simulink model "TestStructure"  (R2022b)
settings: Solver=FixedStepDiscrete  StartTime=0.0  StopTime=300  FixedStep=SampleTime  RelTol=1e-3
InitFcn:
  | SampleTime = 0.001;
  | ButtonValue=0;
  | load("BusConfig.mat");
model workspace (MAT data in the model file):
  Manual_Auto = 1
  Pattern = 1
  Pause_Start = 1
  Stop = 1
  Unlock_Lock = 1
undefined symbols (not defined in the file or in its folder): DiscIntNeverNeededParam
libraries: dspfdesign x4, dspstat3 x4
(part 3 of 3)

== system TestStructure/Control/Tasks/LLBManualTask/Subsystem1/If Action Subsystem2 ==
  Motor1Pos : Inport
  Action Port : ActionPort  ActionPortLabel=if((u1 >= u2))
  Out1 : Outport
  wires:
  Motor1Pos/1 -> Out1/1

== system TestStructure/Control/Tasks/LLBManualTask/Subsystem2/If Action Subsystem4 ==
  In1 : Inport
  Action Port : ActionPort  ActionPortLabel=else
  Out1 : Outport
  wires:
  In1/1 -> Out1/1

== system TestStructure/Control/Tasks/LLBManualTask/Subsystem2/If Action Subsystem5 ==
  In1 : Inport
  Action Port : ActionPort  ActionPortLabel=if((u1 <= u2))
  Out1 : Outport
  wires:
  In1/1 -> Out1/1

== system TestStructure/Control/Tasks/LLBManualTask/Subsystem3/If Action Subsystem1 ==
  In1 : Inport
  Action Port : ActionPort  ActionPortLabel=else
  Out1 : Outport
  wires:
  In1/1 -> Out1/1

== system TestStructure/Control/Tasks/LLBManualTask/Subsystem3/If Action Subsystem2 ==
  Motor1Pos : Inport
  Action Port : ActionPort  ActionPortLabel=if((u1 >= u2))
  Out1 : Outport
  wires:
  Motor1Pos/1 -> Out1/1

== system TestStructure/Control/Tasks/LLWManualTask/Subsystem/If Action Subsystem4 ==
  In1 : Inport
  Action Port : ActionPort  ActionPortLabel=else
  Out1 : Outport
  wires:
  In1/1 -> Out1/1

== system TestStructure/Control/Tasks/LLWManualTask/Subsystem/If Action Subsystem5 ==
  In1 : Inport
  Action Port : ActionPort  ActionPortLabel=if((u1 <= u2))
  Out1 : Outport
  wires:
  In1/1 -> Out1/1

== system TestStructure/Control/Tasks/LLWManualTask/Subsystem1/If Action Subsystem1 ==
  In1 : Inport
  Action Port : ActionPort  ActionPortLabel=else
  Out1 : Outport
  wires:
  In1/1 -> Out1/1

== system TestStructure/Control/Tasks/LLWManualTask/Subsystem1/If Action Subsystem2 ==
  Motor1Pos : Inport
  Action Port : ActionPort  ActionPortLabel=if((u1 >= u2))
  Out1 : Outport
  wires:
  Motor1Pos/1 -> Out1/1

== system TestStructure/Control/Tasks/LLWManualTask/Subsystem2/If Action Subsystem4 ==
  In1 : Inport
  Action Port : ActionPort  ActionPortLabel=else
  Out1 : Outport
  wires:
  In1/1 -> Out1/1

== system TestStructure/Control/Tasks/LLWManualTask/Subsystem2/If Action Subsystem5 ==
  In1 : Inport
  Action Port : ActionPort  ActionPortLabel=if((u1 <= u2))
  Out1 : Outport
  wires:
  In1/1 -> Out1/1

== system TestStructure/Control/Tasks/LLWManualTask/Subsystem3/If Action Subsystem1 ==
  In1 : Inport
  Action Port : ActionPort  ActionPortLabel=else
  Out1 : Outport
  wires:
  In1/1 -> Out1/1

== system TestStructure/Control/Tasks/LLWManualTask/Subsystem3/If Action Subsystem2 ==
  Motor1Pos : Inport
  Action Port : ActionPort  ActionPortLabel=if((u1 >= u2))
  Out1 : Outport
  wires:
  Motor1Pos/1 -> Out1/1

== stateflow chart TestStructure/Control/Tasks/LLBManualTask/RythmModel/Chart ==
  state IntStateOperation
    Count =1/(Period*SampleTime);
    Input=1/Period;
    Reset = 0;
  state ResetOperation
    Reset = 1;
  (default) -> IntStateOperation
  ResetOperation -> IntStateOperation : [IntVal<(Count)*(Period*SampleTime)]
  IntStateOperation -> ResetOperation : [IntVal>=(Count)*(Period*SampleTime)||(ResetState==1)]
  data: ResetState input; Period input; SampleTime input; Input output; Reset output; IntVal input; Count local

== stateflow chart TestStructure/Control/Tasks/LLWManualTask/RythmModel/Chart ==
  state IntStateOperation
    Count =1/(Period*SampleTime);
    Input=1/Period;
    Reset = 0;
  state ResetOperation
    Reset = 1;
  (default) -> IntStateOperation
  ResetOperation -> IntStateOperation : [IntVal<(Count)*(Period*SampleTime)]
  IntStateOperation -> ResetOperation : [IntVal>=(Count)*(Period*SampleTime)||(ResetState==1)]
  data: ResetState input; Period input; SampleTime input; Input output; Reset output; IntVal input; Count local

== stateflow chart TestStructure/Control/PanelController/ControlPannelStateMachine ==
  state Pause
    State = "Pause";
    if(Pause_StartButtonPressed==0)
    Pause_StartButtonPressed_temp = 0;
    end
  state Stop
    (history)
    state Stop
      State = "Stop";
    state LowerLimb_Follow
      state LowerLimb_Follow
        if(PatternButtonPressed==0)
        PatternButtonPressed_temp = 0;
        end
        State = "Stop";
        Mode = "Lower_Limb_Follow";
        ManualAuto = "";
      (default) -> Stop.LowerLimb_Follow.LowerLimb_Follow
    state LowerLimb_FlutterKick
      (history)
      state LowerLimb_FlutterKick
        if(PatternButtonPressed==0)
        PatternButtonPressed_temp = 0;
        end
        State = "Stop";
        Mode = "Lower_Limb_FlutterKick";
      state LLFK_Manual_Torque
        if(PatternButtonPressed==0)
        PatternButtonPressed_temp = 0;
        end
        if(Manual_AutoButtonPressed==0)
        Manual_AutoButtonPressed_temp = 0;
        end
        State = "Stop";
        Mode = "Lower_Limb_FlutterKick";
        ManualAuto = "LLFK_Manual_Torque";
      state LLFK_Manual_Freq
        if(PatternButtonPressed==0)
        PatternButtonPressed_temp = 0;
        end
        if(Manual_AutoButtonPressed==0)
        Manual_AutoButtonPressed_temp = 0;
        end
        State = "Stop";
        Mode = "Lower_Limb_FlutterKick";
        ManualAuto = "LLFK_Manual_Freq";
      state LLFK_Manual_Pos
        if(PatternButtonPressed==0)
        PatternButtonPressed_temp = 0;
        end
        if(Manual_AutoButtonPressed==0)
        Manual_AutoButtonPressed_temp = 0;
        end
        State = "Stop";
        Mode = "Lower_Limb_FlutterKick";
        ManualAuto = "LLFK_Manual_Pos";
      state LLFK_Auto
        if(PatternButtonPressed==0)
        PatternButtonPressed_temp = 0;
        end
        if(Manual_AutoButtonPressed==0)
        Manual_AutoButtonPressed_temp = 0;
        end
        State = "Stop";
        Mode = "Lower_Limb_FlutterKick";
        ManualAuto = "LLFK_Auto";
      (default) -> Stop.LowerLimb_FlutterKick.LowerLimb_FlutterKick
      Stop.LowerLimb_FlutterKick.LowerLimb_FlutterKick -> LLFK_Manual_Freq
      LLFK_Manual_Freq -> LLFK_Manual_Torque : [(Manual_AutoButtonPressed_temp==0)&&(Manual_AutoButtonPressed>0)]{Manual_AutoButtonPressed_temp=1;}
      LLFK_Manual_Torque -> LLFK_Manual_Pos : [(Manual_AutoButtonPressed_temp==0)&&(Manual_AutoButtonPressed>0)]{Manual_AutoButtonPressed_temp=1;}
      LLFK_Auto -> LLFK_Manual_Freq : [(Manual_AutoButtonPressed_temp==0)&&(Manual_AutoButtonPressed>0)]{Manual_AutoButtonPressed_temp=1;}
      LLFK_Manual_Pos -> LLFK_Auto : [(Manual_AutoButtonPressed_temp==0)&&(Manual_AutoButtonPressed>0)]{Manual_AutoButtonPressed_temp=1;}
    state LowerLimb_Breaststroke
      (history)
      state Lower_Limb_Breaststroke
        if(PatternButtonPressed==0)
        PatternButtonPressed_temp = 0;
        end
        State = "Stop";
        Mode = "Lower_Limb_Breaststroke";
      state LLB_Manual_Torque
        if(PatternButtonPressed==0)
        PatternButtonPressed_temp = 0;
        end
        if(Manual_AutoButtonPressed==0)
        Manual_AutoButtonPressed_temp = 0;
        end
        State = "Stop";
        Mode = "Lower_Limb_Breaststroke";
        ManualAuto = "LLB_Manual_Torque";
      state LLB_Manual_Freq
        if(PatternButtonPressed==0)
        PatternButtonPressed_temp = 0;
        end
        if(Manual_AutoButtonPressed==0)
        Manual_AutoButtonPressed_temp = 0;
        end
        State = "Stop";
        Mode = "Lower_Limb_Breaststroke";
        ManualAuto = "LLB_Manual_Freq";
      state LLB_Manual_Pos
        if(PatternButtonPressed==0)
        PatternButtonPressed_temp = 0;
        end
        if(Manual_AutoButtonPressed==0)
        Manual_AutoButtonPressed_temp = 0;
        end
        State = "Stop";
        Mode = "Lower_Limb_Breaststroke";
        ManualAuto = "LLB_Manual_Pos";
      state LLB_Auto
        if(PatternButtonPressed==0)
        PatternButtonPressed_temp = 0;
        end
        if(Manual_AutoButtonPressed==0)
        Manual_AutoButtonPressed_temp = 0;
        end
        State = "Stop";
        Mode = "Lower_Limb_Breaststroke";
        ManualAuto = "LLB_Auto";
      (default) -> Lower_Limb_Breaststroke
      Lower_Limb_Breaststroke -> LLB_Manual_Freq
      LLB_Manual_Freq -> LLB_Manual_Torque : [(Manual_AutoButtonPressed_temp==0)&&(Manual_AutoButtonPressed>0)]{Manual_AutoButtonPressed_temp=1;}
      LLB_Manual_Torque -> LLB_Manual_Pos : [(Manual_AutoButtonPressed_temp==0)&&(Manual_AutoButtonPressed>0)]{Manual_AutoButtonPressed_temp=1;}
      LLB_Auto -> LLB_Manual_Freq : [(Manual_AutoButtonPressed_temp==0)&&(Manual_AutoButtonPressed>0)]{Manual_AutoButtonPressed_temp=1;}
      LLB_Manual_Pos -> LLB_Auto : [(Manual_AutoButtonPressed_temp==0)&&(Manual_AutoButtonPressed>0)]{Manual_AutoButtonPressed_temp=1;}
    state LowerLimb_Walk
      (history)
      state LowerLimb_Walk
        if(PatternButtonPressed==0)
        PatternButtonPressed_temp = 0;
        end
        State = "Stop";
        Mode = "Lower_Limb_Walk";
      state LLW_Manual_Torque
        if(PatternButtonPressed==0)
        PatternButtonPressed_temp = 0;
        end
        if(Manual_AutoButtonPressed==0)
        Manual_AutoButtonPressed_temp = 0;
        end
        State = "Stop";
        Mode = "Lower_Limb_Walk";
        ManualAuto = "LLW_Manual_Torque";
      state LLW_Manual_Freq
        if(PatternButtonPressed==0)
        PatternButtonPressed_temp = 0;
        end
        if(Manual_AutoButtonPressed==0)
        Manual_AutoButtonPressed_temp = 0;
        end
        State = "Stop";
        Mode = "Lower_Limb_Walk";
        ManualAuto = "LLW_Manual_Freq";
      state LLW_Manual_Pos
        if(PatternButtonPressed==0)
        PatternButtonPressed_temp = 0;
        end
        if(Manual_AutoButtonPressed==0)
        Manual_AutoButtonPressed_temp = 0;
        end
        State = "Stop";
        Mode = "Lower_Limb_Walk";
        ManualAuto = "LLW_Manual_Pos";
      state LLW_Auto
        if(PatternButtonPressed==0)
        PatternButtonPressed_temp = 0;
        end
        if(Manual_AutoButtonPressed==0)
        Manual_AutoButtonPressed_temp = 0;
        end
        State = "Stop";
        Mode = "Lower_Limb_Walk";
        ManualAuto = "LLW_Auto";
      (default) -> Stop.LowerLimb_Walk.LowerLimb_Walk
      Stop.LowerLimb_Walk.LowerLimb_Walk -> LLW_Manual_Freq
      LLW_Manual_Freq -> LLW_Manual_Torque : [(Manual_AutoButtonPressed_temp==0)&&(Manual_AutoButtonPressed>0)]{Manual_AutoButtonPressed_temp=1;}
      LLW_Manual_Torque -> LLW_Manual_Pos : [(Manual_AutoButtonPressed_temp==0)&&(Manual_AutoButtonPressed>0)]{Manual_AutoButtonPressed_temp=1;}
      LLW_Auto -> LLW_Manual_Freq : [(Manual_AutoButtonPressed_temp==0)&&(Manual_AutoButtonPressed>0)]{Manual_AutoButtonPressed_temp=1;}
      LLW_Manual_Pos -> LLW_Auto : [(Manual_AutoButtonPressed_temp==0)&&(Manual_AutoButtonPressed>0)]{Manual_AutoButtonPressed_temp=1;}
    (default) -> Stop.Stop
    Stop.Stop -> Stop.LowerLimb_Follow
    Stop.LowerLimb_Follow -> Stop.LowerLimb_FlutterKick : [(PatternButtonPressed_temp==0)&&(PatternButtonPressed>0)]{PatternButtonPressed_temp=1;}
    LowerLimb_Breaststroke -> Stop.LowerLimb_Walk : [(PatternButtonPressed_temp==0)&&(PatternButtonPressed>0)]{PatternButtonPressed_temp=1;}
    Stop.LowerLimb_FlutterKick -> LowerLimb_Breaststroke : [(PatternButtonPressed_temp==0)&&(PatternButtonPressed>0)]{PatternButtonPressed_temp=1;}
    Stop.LowerLimb_Walk -> Stop.LowerLimb_Follow : [(PatternButtonPressed_temp==0)&&(PatternButtonPressed>0)]{PatternButtonPressed_temp=1;}
  state Start
    state Start
      State = "Start";
      if(Pause_StartButtonPressed==0)
      Pause_StartButtonPressed_temp = 0;
      end
    state UpperLimb_Lock
      if(Pause_StartButtonPressed==0)
      Pause_StartButtonPressed_temp = 0;
      end
      if(Unlock_LockButtonPressed==0)
      Unlock_LockButtonPressed_temp = 0;
      end
      State = "Start";
      UnlockLock = "UpperLimb_Lock";
    state UpperLimb_UnLock
      if(Pause_StartButtonPressed==0)
      Pause_StartButtonPressed_temp = 0;
      end
      if(Unlock_LockButtonPressed==0)
      Unlock_LockButtonPressed_temp = 0;
      end
      State = "Start";
      UnlockLock = "UpperLimb_Unlock";
    (default) -> Start.Start
    Start.Start -> UpperLimb_UnLock
    UpperLimb_Lock -> UpperLimb_UnLock : [(Unlock_LockButtonPressed_temp==0)&&(Unlock_LockButtonPressed>0)]{Unlock_LockButtonPressed_temp=1;}
    UpperLimb_UnLock -> UpperLimb_Lock : [(Unlock_LockButtonPressed_temp==0)&&(Unlock_LockButtonPressed>0)]{Unlock_LockButtonPressed_temp=1;}
  Start -> Pause : [(Pause_StartButtonPressed_temp==0)&&(Pause_StartButtonPressed>0)]{Pause_StartButtonPressed_temp=1;UnlockLock = "UpperLimb_Unlock";}
  Pause -> Stop [order 2] : [StopButtonPressed>0]
  Pause -> Start [order 1] : [(Pause_StartButtonPressed_temp==0)&&(Pause_StartButtonPressed>0)&&(TaskFinished==9)]{Pause_StartButtonPressed_temp=1;}
  (default) -> Stop
  Stop -> Start : [(Pause_StartButtonPressed>0)&&(TaskFinished==1)]{Pause_StartButtonPressed_temp=1;}
  data: TaskFinished input; StopButtonPressed input; State output; Pause_StartButtonPressed input; Pause_StartButtonPressed_temp local; PatternButtonPressed input; Manual_AutoButtonPressed input; Manual_AutoButtonPressed_temp local; PatternButtonPressed_temp local; Mode output string; ManualAuto output string; UnlockLock output string; Unlock_LockButtonPressed input; Unlock_LockButtonPressed_temp local

== stateflow chart TestStructure/Control/PanelController/KnobStateMachine ==
  state Start
    kState = "Start";
  state Adjust
    state LLF_Adjust
    state Adjust
      kState = "Adjust";
    state LLFK_Adjust
      state LLFK_Auto
      state LLFK_Adjust
        kState = "LLFK_Adjust";
      state LLFK_Freq_Adjust
        state LLFK_Freq_Adjust
          kState = "LLFK_Freq";
          LLFK_Freq = 0;
          LLFK_Torque_Up = 0;
          LLFK_Torque_Down = 0;
          LLFK_Pos_Up = 0;
          LLFK_Pos_Down = 0;
          LLB_Freq = 0;
          LLB_Torque_Up = 0;
          LLB_Torque_Down = 0;
          LLB_Pos_Up = 0;
          LLB_Pos_Down = 0;
          LLW_Freq = 0;
          LLW_Torque_Up = 0;
          LLW_Torque_Down = 0;
          LLW_Pos_Up = 0;
          LLW_Pos_Down = 0;
          Freq_Up_temp = 0;
          Freq_Down_temp = 0;
        state Freq_Up
          if(Freq_Up==0)
          Freq_Up_temp = 0;
          LLFK_Freq = 1;
          end
        state Freq_Down
          if(Freq_Down==0)
          Freq_Down_temp = 0;
          LLFK_Freq = -1;
          end
        (default) -> Adjust.LLFK_Adjust.LLFK_Freq_Adjust.LLFK_Freq_Adjust
        Adjust.LLFK_Adjust.LLFK_Freq_Adjust.LLFK_Freq_Adjust -> Adjust.LLFK_Adjust.LLFK_Freq_Adjust.Freq_Down [order 2] : [(Freq_Down_temp==0)&&(Freq_Down>0)]{Freq_Down_temp=1;}
        Adjust.LLFK_Adjust.LLFK_Freq_Adjust.LLFK_Freq_Adjust -> Adjust.LLFK_Adjust.LLFK_Freq_Adjust.Freq_Up [order 1] : [(Freq_Up_temp==0)&&(Freq_Up>0)]{Freq_Up_temp=1;}
        Adjust.LLFK_Adjust.LLFK_Freq_Adjust.Freq_Up -> Adjust.LLFK_Adjust.LLFK_Freq_Adjust.LLFK_Freq_Adjust : [Freq_Up_temp == 0]
        Adjust.LLFK_Adjust.LLFK_Freq_Adjust.Freq_Down -> Adjust.LLFK_Adjust.LLFK_Freq_Adjust.LLFK_Freq_Adjust : [Freq_Down_temp == 0]
      state LLFK_Torque_Adjust
        state Negtive_Up
          if(Negtive_Up==0)
          Negtive_Up_temp = 0;
          LLFK_Torque_Down = 1;
          end
        state LLFK_Torque_Adjust
          kState = "LLFK_Torq";
          LLFK_Freq = 0;
          LLFK_Torque_Up = 0;
          LLFK_Torque_Down = 0;
          LLFK_Pos_Up = 0;
          LLFK_Pos_Down = 0;
          LLB_Freq = 0;
          LLB_Torque_Up = 0;
          LLB_Torque_Down = 0;
          LLB_Pos_Up = 0;
          LLB_Pos_Down = 0;
          LLW_Freq = 0;
          LLW_Torque_Up = 0;
          LLW_Torque_Down = 0;
          LLW_Pos_Up = 0;
          LLW_Pos_Down = 0;
          Negtive_Up_temp = 0;
          Negtive_Down_temp = 0;
          Positive_Up_temp = 0;
          Positive_Down_temp = 0;
        state Negtive_Down
          if(Negtive_Down==0)
          Negtive_Down_temp = 0;
          LLFK_Torque_Down = -1;
          end
        state Positive_Up
          if(Positive_Up==0)
          Positive_Up_temp = 0;
          LLFK_Torque_Up = 1;
          end
        state Positive_Down
          if(Positive_Down==0)
          Positive_Down_temp = 0;
          LLFK_Torque_Up = -1;
          end
        (default) -> Adjust.LLFK_Adjust.LLFK_Torque_Adjust.LLFK_Torque_Adjust
        Adjust.LLFK_Adjust.LLFK_Torque_Adjust.LLFK_Torque_Adjust -> Adjust.LLFK_Adjust.LLFK_Torque_Adjust.Negtive_Up [order 4] : [(Negtive_Up_temp==0)&&(Negtive_Up>0)]{Negtive_Up_temp=1;}
        Adjust.LLFK_Adjust.LLFK_Torque_Adjust.LLFK_Torque_Adjust -> Adjust.LLFK_Adjust.LLFK_Torque_Adjust.Negtive_Down [order 2] : [(Negtive_Down_temp==0)&&(Negtive_Down>0)]{Negtive_Down_temp=1;}
        Adjust.LLFK_Adjust.LLFK_Torque_Adjust.Negtive_Down -> Adjust.LLFK_Adjust.LLFK_Torque_Adjust.LLFK_Torque_Adjust : [Negtive_Down_temp == 0]
        Adjust.LLFK_Adjust.LLFK_Torque_Adjust.Negtive_Up -> Adjust.LLFK_Adjust.LLFK_Torque_Adjust.LLFK_Torque_Adjust : [Negtive_Up_temp == 0]
        Adjust.LLFK_Adjust.LLFK_Torque_Adjust.LLFK_Torque_Adjust -> Adjust.LLFK_Adjust.LLFK_Torque_Adjust.Positive_Up [order 3] : [(Positive_Up_temp==0)&&(Positive_Up>0)]{Positive_Up_temp=1;}
        Adjust.LLFK_Adjust.LLFK_Torque_Adjust.LLFK_Torque_Adjust -> Adjust.LLFK_Adjust.LLFK_Torque_Adjust.Positive_Down [order 1] : [(Positive_Down_temp==0)&&(Positive_Down>0)]{Positive_Down_temp=1;}
        Adjust.LLFK_Adjust.LLFK_Torque_Adjust.Positive_Up -> Adjust.LLFK_Adjust.LLFK_Torque_Adjust.LLFK_Torque_Adjust : [Positive_Up_temp == 0]
        Adjust.LLFK_Adjust.LLFK_Torque_Adjust.Positive_Down -> Adjust.LLFK_Adjust.LLFK_Torque_Adjust.LLFK_Torque_Adjust : [Positive_Down_temp == 0]
      state LLFK_Pos_Adjust
        state Negtive_Up
          if(Negtive_Up==0)
          Negtive_Up_temp = 0;
          LLFK_Pos_Down = 1;
          end
        state LLFK_Pos_Adjust
          kState = "LLFK_Pos";
          LLFK_Freq = 0;
          LLFK_Torque_Up = 0;
          LLFK_Torque_Down = 0;
          LLFK_Pos_Up = 0;
          LLFK_Pos_Down = 0;
          LLB_Freq = 0;
          LLB_Torque_Up = 0;
          LLB_Torque_Down = 0;
          LLB_Pos_Up = 0;
          LLB_Pos_Down = 0;
          LLW_Freq = 0;
          LLW_Torque_Up = 0;
          LLW_Torque_Down = 0;
          LLW_Pos_Up = 0;
          LLW_Pos_Down = 0;
          Negtive_Up_temp = 0;
          Negtive_Down_temp = 0;
          Positive_Up_temp = 0;
          Positive_Down_temp = 0;
        state Negtive_Down
          if(Negtive_Down==0)
          Negtive_Down_temp = 0;
          LLFK_Pos_Down = -1;
          end
        state Positive_Up
          if(Positive_Up==0)
          Positive_Up_temp = 0;
          LLFK_Pos_Up = 1;
          end
        state Positive_Down
          if(Positive_Down==0)
          Positive_Down_temp = 0;
          LLFK_Pos_Up = -1;
          end
        (default) -> Adjust.LLFK_Adjust.LLFK_Pos_Adjust.LLFK_Pos_Adjust
        Adjust.LLFK_Adjust.LLFK_Pos_Adjust.LLFK_Pos_Adjust -> Adjust.LLFK_Adjust.LLFK_Pos_Adjust.Negtive_Up [order 4] : [(Negtive_Up_temp==0)&&(Negtive_Up>0)]{Negtive_Up_temp=1;}
        Adjust.LLFK_Adjust.LLFK_Pos_Adjust.LLFK_Pos_Adjust -> Adjust.LLFK_Adjust.LLFK_Pos_Adjust.Negtive_Down [order 2] : [(Negtive_Down_temp==0)&&(Negtive_Down>0)]{Negtive_Down_temp=1;}
        Adjust.LLFK_Adjust.LLFK_Pos_Adjust.Negtive_Down -> Adjust.LLFK_Adjust.LLFK_Pos_Adjust.LLFK_Pos_Adjust : [Negtive_Down_temp == 0]
        Adjust.LLFK_Adjust.LLFK_Pos_Adjust.Negtive_Up -> Adjust.LLFK_Adjust.LLFK_Pos_Adjust.LLFK_Pos_Adjust : [Negtive_Up_temp == 0]
        Adjust.LLFK_Adjust.LLFK_Pos_Adjust.LLFK_Pos_Adjust -> Adjust.LLFK_Adjust.LLFK_Pos_Adjust.Positive_Up [order 3] : [(Positive_Up_temp==0)&&(Positive_Up>0)]{Positive_Up_temp=1;}
        Adjust.LLFK_Adjust.LLFK_Pos_Adjust.LLFK_Pos_Adjust -> Adjust.LLFK_Adjust.LLFK_Pos_Adjust.Positive_Down [order 1] : [(Positive_Down_temp==0)&&(Positive_Down>0)]{Positive_Down_temp=1;}
        Adjust.LLFK_Adjust.LLFK_Pos_Adjust.Positive_Up -> Adjust.LLFK_Adjust.LLFK_Pos_Adjust.LLFK_Pos_Adjust : [Positive_Up_temp == 0]
        Adjust.LLFK_Adjust.LLFK_Pos_Adjust.Positive_Down -> Adjust.LLFK_Adjust.LLFK_Pos_Adjust.LLFK_Pos_Adjust : [Positive_Down_temp == 0]
      Adjust.LLFK_Adjust.LLFK_Adjust -> LLFK_Auto [order 4] : [ManualAuto=="LLFK_Auto"]{Display_State=1;}
      LLFK_Auto -> Adjust.LLFK_Adjust.LLFK_Adjust : [ManualAuto~="LLFK_Auto"]{Display_State=2;}
      (default) -> Adjust.LLFK_Adjust.LLFK_Adjust
      Adjust.LLFK_Adjust.LLFK_Pos_Adjust -> Adjust.LLFK_Adjust.LLFK_Adjust : [ManualAuto~="LLFK_Manual_Pos"]
      Adjust.LLFK_Adjust.LLFK_Adjust -> Adjust.LLFK_Adjust.LLFK_Freq_Adjust [order 3] : [ManualAuto=="LLFK_Manual_Freq"]
      Adjust.LLFK_Adjust.LLFK_Freq_Adjust -> Adjust.LLFK_Adjust.LLFK_Adjust : [ManualAuto~="LLFK_Manual_Freq"]
      Adjust.LLFK_Adjust.LLFK_Adjust -> Adjust.LLFK_Adjust.LLFK_Pos_Adjust [order 1] : [ManualAuto=="LLFK_Manual_Pos"]
      Adjust.LLFK_Adjust.LLFK_Adjust -> Adjust.LLFK_Adjust.LLFK_Torque_Adjust [order 2] : [ManualAuto=="LLFK_Manual_Torque"]
      Adjust.LLFK_Adjust.LLFK_Torque_Adjust -> Adjust.LLFK_Adjust.LLFK_Adjust : [ManualAuto~="LLFK_Manual_Torque"]
    state LLB_Adjust
      state LLB_Auto
      state LLB_Adjust
        kState = "LLB_Adjust";
      state LLB_Freq_Adjust
        state LLB_Freq_Adjust
          kState = "LLB_Freq";
          LLFK_Freq = 0;
          LLFK_Torque_Up = 0;
          LLFK_Torque_Down = 0;
          LLFK_Pos_Up = 0;
          LLFK_Pos_Down = 0;
          LLB_Freq = 0;
          LLB_Torque_Up = 0;
          LLB_Torque_Down = 0;
          LLB_Pos_Up = 0;
          LLB_Pos_Down = 0;
          LLW_Freq = 0;
          LLW_Torque_Up = 0;
          LLW_Torque_Down = 0;
          LLW_Pos_Up = 0;
          LLW_Pos_Down = 0;
          Freq_Up_temp = 0;
          Freq_Down_temp = 0;
        state Freq_Up
          if(Freq_Up==0)
          Freq_Up_temp = 0;
          LLB_Freq = 1;
          end
        state Freq_Down
          if(Freq_Down==0)
          Freq_Down_temp = 0;
          LLB_Freq = -1;
          end
        (default) -> Adjust.LLB_Adjust.LLB_Freq_Adjust.LLB_Freq_Adjust
        Adjust.LLB_Adjust.LLB_Freq_Adjust.LLB_Freq_Adjust -> Adjust.LLB_Adjust.LLB_Freq_Adjust.Freq_Down [order 2] : [(Freq_Down_temp==0)&&(Freq_Down>0)]{Freq_Down_temp=1;}
        Adjust.LLB_Adjust.LLB_Freq_Adjust.LLB_Freq_Adjust -> Adjust.LLB_Adjust.LLB_Freq_Adjust.Freq_Up [order 1] : [(Freq_Up_temp==0)&&(Freq_Up>0)]{Freq_Up_temp=1;}
        Adjust.LLB_Adjust.LLB_Freq_Adjust.Freq_Up -> Adjust.LLB_Adjust.LLB_Freq_Adjust.LLB_Freq_Adjust : [Freq_Up_temp == 0]
        Adjust.LLB_Adjust.LLB_Freq_Adjust.Freq_Down -> Adjust.LLB_Adjust.LLB_Freq_Adjust.LLB_Freq_Adjust : [Freq_Down_temp == 0]
      state LLB_Torque_Adjust
        state Negtive_Up
          if(Negtive_Up==0)
          Negtive_Up_temp = 0;
          LLB_Torque_Down = 1;
          end
        state LLB_Torque_Adjust
          kState = "LLB_Torq";
          LLFK_Freq = 0;
          LLFK_Torque_Up = 0;
          LLFK_Torque_Down = 0;
          LLFK_Pos_Up = 0;
          LLFK_Pos_Down = 0;
          LLB_Freq = 0;
          LLB_Torque_Up = 0;
          LLB_Torque_Down = 0;
          LLB_Pos_Up = 0;
          LLB_Pos_Down = 0;
          LLW_Freq = 0;
          LLW_Torque_Up = 0;
          LLW_Torque_Down = 0;
          LLW_Pos_Up = 0;
          LLW_Pos_Down = 0;
          Negtive_Up_temp = 0;
          Negtive_Down_temp = 0;
          Positive_Up_temp = 0;
          Positive_Down_temp = 0;
        state Negtive_Down
          if(Negtive_Down==0)
          Negtive_Down_temp = 0;
          LLB_Torque_Down = -1;
          end
        state Positive_Up
          if(Positive_Up==0)
          Positive_Up_temp = 0;
          LLB_Torque_Up = 1;
          end
        state Positive_Down
          if(Positive_Down==0)
          Positive_Down_temp = 0;
          LLB_Torque_Up = -1;
          end
        (default) -> Adjust.LLB_Adjust.LLB_Torque_Adjust.LLB_Torque_Adjust
        Adjust.LLB_Adjust.LLB_Torque_Adjust.LLB_Torque_Adjust -> Adjust.LLB_Adjust.LLB_Torque_Adjust.Negtive_Up [order 4] : [(Negtive_Up_temp==0)&&(Negtive_Up>0)]{Negtive_Up_temp=1;}
        Adjust.LLB_Adjust.LLB_Torque_Adjust.LLB_Torque_Adjust -> Adjust.LLB_Adjust.LLB_Torque_Adjust.Negtive_Down [order 2] : [(Negtive_Down_temp==0)&&(Negtive_Down>0)]{Negtive_Down_temp=1;}
        Adjust.LLB_Adjust.LLB_Torque_Adjust.Negtive_Down -> Adjust.LLB_Adjust.LLB_Torque_Adjust.LLB_Torque_Adjust : [Negtive_Down_temp == 0]
        Adjust.LLB_Adjust.LLB_Torque_Adjust.Negtive_Up -> Adjust.LLB_Adjust.LLB_Torque_Adjust.LLB_Torque_Adjust : [Negtive_Up_temp == 0]
        Adjust.LLB_Adjust.LLB_Torque_Adjust.LLB_Torque_Adjust -> Adjust.LLB_Adjust.LLB_Torque_Adjust.Positive_Down [order 1] : [(Positive_Down_temp==0)&&(Positive_Down>0)]{Positive_Down_temp=1;}
        Adjust.LLB_Adjust.LLB_Torque_Adjust.LLB_Torque_Adjust -> Adjust.LLB_Adjust.LLB_Torque_Adjust.Positive_Up [order 3] : [(Positive_Up_temp==0)&&(Positive_Up>0)]{Positive_Up_temp=1;}
        Adjust.LLB_Adjust.LLB_Torque_Adjust.Positive_Up -> Adjust.LLB_Adjust.LLB_Torque_Adjust.LLB_Torque_Adjust : [Positive_Up_temp == 0]
        Adjust.LLB_Adjust.LLB_Torque_Adjust.Positive_Down -> Adjust.LLB_Adjust.LLB_Torque_Adjust.LLB_Torque_Adjust : [Positive_Down_temp == 0]
      state LLB_Pos_Adjust
        state Negtive_Up
          if(Negtive_Up==0)
          Negtive_Up_temp = 0;
          LLB_Pos_Down = 1;
          end
        state LLB_Pos_Adjust
          kState = "LLB_Pos";
          LLFK_Freq = 0;
          LLFK_Torque_Up = 0;
          LLFK_Torque_Down = 0;
          LLFK_Pos_Up = 0;
          LLFK_Pos_Down = 0;
          LLB_Freq = 0;
          LLB_Torque_Up = 0;
          LLB_Torque_Down = 0;
          LLB_Pos_Up = 0;
          LLB_Pos_Down = 0;
          LLW_Freq = 0;
          LLW_Torque_Up = 0;
          LLW_Torque_Down = 0;
          LLW_Pos_Up = 0;
          LLW_Pos_Down = 0;
          Negtive_Up_temp = 0;
          Negtive_Down_temp = 0;
          Positive_Up_temp = 0;
          Positive_Down_temp = 0;
        state Negtive_Down
          if(Negtive_Down==0)
          Negtive_Down_temp = 0;
          LLB_Pos_Down = -1;
          end
        state Positive_Up
          if(Positive_Up==0)
          Positive_Up_temp = 0;
          LLB_Pos_Up = 1;
          end
        state Positive_Down
          if(Positive_Down==0)
          Positive_Down_temp = 0;
          LLB_Pos_Up = -1;
          end
        (default) -> Adjust.LLB_Adjust.LLB_Pos_Adjust.LLB_Pos_Adjust
        Adjust.LLB_Adjust.LLB_Pos_Adjust.LLB_Pos_Adjust -> Adjust.LLB_Adjust.LLB_Pos_Adjust.Negtive_Up [order 4] : [(Negtive_Up_temp==0)&&(Negtive_Up>0)]{Negtive_Up_temp=1;}
        Adjust.LLB_Adjust.LLB_Pos_Adjust.LLB_Pos_Adjust -> Adjust.LLB_Adjust.LLB_Pos_Adjust.Negtive_Down [order 2] : [(Negtive_Down_temp==0)&&(Negtive_Down>0)]{Negtive_Down_temp=1;}
        Adjust.LLB_Adjust.LLB_Pos_Adjust.Negtive_Down -> Adjust.LLB_Adjust.LLB_Pos_Adjust.LLB_Pos_Adjust : [Negtive_Down_temp == 0]
        Adjust.LLB_Adjust.LLB_Pos_Adjust.Negtive_Up -> Adjust.LLB_Adjust.LLB_Pos_Adjust.LLB_Pos_Adjust : [Negtive_Up_temp == 0]
        Adjust.LLB_Adjust.LLB_Pos_Adjust.LLB_Pos_Adjust -> Adjust.LLB_Adjust.LLB_Pos_Adjust.Positive_Up [order 3] : [(Positive_Up_temp==0)&&(Positive_Up>0)]{Positive_Up_temp=1;}
        Adjust.LLB_Adjust.LLB_Pos_Adjust.LLB_Pos_Adjust -> Adjust.LLB_Adjust.LLB_Pos_Adjust.Positive_Down [order 1] : [(Positive_Down_temp==0)&&(Positive_Down>0)]{Positive_Down_temp=1;}
        Adjust.LLB_Adjust.LLB_Pos_Adjust.Positive_Up -> Adjust.LLB_Adjust.LLB_Pos_Adjust.LLB_Pos_Adjust : [Positive_Up_temp == 0]
        Adjust.LLB_Adjust.LLB_Pos_Adjust.Positive_Down -> Adjust.LLB_Adjust.LLB_Pos_Adjust.LLB_Pos_Adjust : [Positive_Down_temp == 0]
      Adjust.LLB_Adjust.LLB_Adjust -> LLB_Auto [order 4] : [ManualAuto=="LLB_Auto"]{Display_State=1;}
      LLB_Auto -> Adjust.LLB_Adjust.LLB_Adjust : [ManualAuto~="LLB_Auto"]{Display_State=3;}
      (default) -> Adjust.LLB_Adjust.LLB_Adjust
      Adjust.LLB_Adjust.LLB_Pos_Adjust -> Adjust.LLB_Adjust.LLB_Adjust : [ManualAuto~="LLB_Manual_Pos"]
      Adjust.LLB_Adjust.LLB_Adjust -> Adjust.LLB_Adjust.LLB_Freq_Adjust [order 3] : [ManualAuto=="LLB_Manual_Freq"]
      Adjust.LLB_Adjust.LLB_Freq_Adjust -> Adjust.LLB_Adjust.LLB_Adjust : [ManualAuto~="LLB_Manual_Freq"]
      Adjust.LLB_Adjust.LLB_Adjust -> Adjust.LLB_Adjust.LLB_Pos_Adjust [order 1] : [ManualAuto=="LLB_Manual_Pos"]
      Adjust.LLB_Adjust.LLB_Adjust -> Adjust.LLB_Adjust.LLB_Torque_Adjust [order 2] : [ManualAuto=="LLB_Manual_Torque"]
      Adjust.LLB_Adjust.LLB_Torque_Adjust -> Adjust.LLB_Adjust.LLB_Adjust : [ManualAuto~="LLB_Manual_Torque"]
    state LLW_Adjust
      state LLW_Auto
      state LLW_Adjust
        kState = "LLW_Adjust";
      state LLW_Freq_Adjust
        state LLW_Freq_Adjust
          kState = "LLW_Freq";
          LLFK_Freq = 0;
          LLFK_Torque_Up = 0;
          LLFK_Torque_Down = 0;
          LLFK_Pos_Up = 0;
          LLFK_Pos_Down = 0;
          LLB_Freq = 0;
          LLB_Torque_Up = 0;
          LLB_Torque_Down = 0;
          LLB_Pos_Up = 0;
          LLB_Pos_Down = 0;
          LLW_Freq = 0;
          LLW_Torque_Up = 0;
          LLW_Torque_Down = 0;
          LLW_Pos_Up = 0;
          LLW_Pos_Down = 0;
          Freq_Up_temp = 0;
          Freq_Down_temp = 0;
        state Freq_Up
          if(Freq_Up==0)
          Freq_Up_temp = 0;
          LLW_Freq = 1;
          end
        state Freq_Down
          if(Freq_Down==0)
          Freq_Down_temp = 0;
          LLW_Freq = -1;
          end
        (default) -> Adjust.LLW_Adjust.LLW_Freq_Adjust.LLW_Freq_Adjust
        Adjust.LLW_Adjust.LLW_Freq_Adjust.LLW_Freq_Adjust -> Adjust.LLW_Adjust.LLW_Freq_Adjust.Freq_Down [order 2] : [(Freq_Down_temp==0)&&(Freq_Down>0)]{Freq_Down_temp=1;}
        Adjust.LLW_Adjust.LLW_Freq_Adjust.LLW_Freq_Adjust -> Adjust.LLW_Adjust.LLW_Freq_Adjust.Freq_Up [order 1] : [(Freq_Up_temp==0)&&(Freq_Up>0)]{Freq_Up_temp=1;}
        Adjust.LLW_Adjust.LLW_Freq_Adjust.Freq_Up -> Adjust.LLW_Adjust.LLW_Freq_Adjust.LLW_Freq_Adjust : [Freq_Up_temp == 0]
        Adjust.LLW_Adjust.LLW_Freq_Adjust.Freq_Down -> Adjust.LLW_Adjust.LLW_Freq_Adjust.LLW_Freq_Adjust : [Freq_Down_temp == 0]
      state LLW_Torque_Adjust
        state Negtive_Up
          if(Negtive_Up==0)
          Negtive_Up_temp = 0;
          LLW_Torque_Down = 1;
          end
        state LLW_Torque_Adjust
          kState = "LLW_Torq";
          LLFK_Freq = 0;
          LLFK_Torque_Up = 0;
          LLFK_Torque_Down = 0;
          LLFK_Pos_Up = 0;
          LLFK_Pos_Down = 0;
          LLB_Freq = 0;
          LLB_Torque_Up = 0;
          LLB_Torque_Down = 0;
          LLB_Pos_Up = 0;
          LLB_Pos_Down = 0;
          LLW_Freq = 0;
          LLW_Torque_Up = 0;
          LLW_Torque_Down = 0;
          LLW_Pos_Up = 0;
          LLW_Pos_Down = 0;
          Negtive_Up_temp = 0;
          Negtive_Down_temp = 0;
          Positive_Up_temp = 0;
          Positive_Down_temp = 0;
        state Negtive_Down
          if(Negtive_Down==0)
          Negtive_Down_temp = 0;
          LLW_Torque_Down = -1;
          end
        state Positive_Up
          if(Positive_Up==0)
          Positive_Up_temp = 0;
          LLW_Torque_Up = 1;
          end
        state Positive_Down
          if(Positive_Down==0)
          Positive_Down_temp = 0;
          LLW_Torque_Up = -1;
          end
        (default) -> Adjust.LLW_Adjust.LLW_Torque_Adjust.LLW_Torque_Adjust
        Adjust.LLW_Adjust.LLW_Torque_Adjust.LLW_Torque_Adjust -> Adjust.LLW_Adjust.LLW_Torque_Adjust.Negtive_Up [order 4] : [(Negtive_Up_temp==0)&&(Negtive_Up>0)]{Negtive_Up_temp=1;}
        Adjust.LLW_Adjust.LLW_Torque_Adjust.LLW_Torque_Adjust -> Adjust.LLW_Adjust.LLW_Torque_Adjust.Negtive_Down [order 2] : [(Negtive_Down_temp==0)&&(Negtive_Down>0)]{Negtive_Down_temp=1;}
        Adjust.LLW_Adjust.LLW_Torque_Adjust.Negtive_Down -> Adjust.LLW_Adjust.LLW_Torque_Adjust.LLW_Torque_Adjust : [Negtive_Down_temp == 0]
        Adjust.LLW_Adjust.LLW_Torque_Adjust.Negtive_Up -> Adjust.LLW_Adjust.LLW_Torque_Adjust.LLW_Torque_Adjust : [Negtive_Up_temp == 0]
        Adjust.LLW_Adjust.LLW_Torque_Adjust.LLW_Torque_Adjust -> Adjust.LLW_Adjust.LLW_Torque_Adjust.Positive_Down [order 1] : [(Positive_Down_temp==0)&&(Positive_Down>0)]{Positive_Down_temp=1;}
        Adjust.LLW_Adjust.LLW_Torque_Adjust.LLW_Torque_Adjust -> Adjust.LLW_Adjust.LLW_Torque_Adjust.Positive_Up [order 3] : [(Positive_Up_temp==0)&&(Positive_Up>0)]{Positive_Up_temp=1;}
        Adjust.LLW_Adjust.LLW_Torque_Adjust.Positive_Up -> Adjust.LLW_Adjust.LLW_Torque_Adjust.LLW_Torque_Adjust : [Positive_Up_temp == 0]
        Adjust.LLW_Adjust.LLW_Torque_Adjust.Positive_Down -> Adjust.LLW_Adjust.LLW_Torque_Adjust.LLW_Torque_Adjust : [Positive_Down_temp == 0]
      state LLW_Pos_Adjust
        state Negtive_Up
          if(Negtive_Up==0)
          Negtive_Up_temp = 0;
          LLW_Pos_Down = 1;
          end
        state LLW_Pos_Adjust
          kState = "LLW_Pos";
          LLFK_Freq = 0;
          LLFK_Torque_Up = 0;
          LLFK_Torque_Down = 0;
          LLFK_Pos_Up = 0;
          LLFK_Pos_Down = 0;
          LLB_Freq = 0;
          LLB_Torque_Up = 0;
          LLB_Torque_Down = 0;
          LLB_Pos_Up = 0;
          LLB_Pos_Down = 0;
          LLW_Freq = 0;
          LLW_Torque_Up = 0;
          LLW_Torque_Down = 0;
          LLW_Pos_Up = 0;
          LLW_Pos_Down = 0;
          Negtive_Up_temp = 0;
          Negtive_Down_temp = 0;
          Positive_Up_temp = 0;
          Positive_Down_temp = 0;
        state Negtive_Down
          if(Negtive_Down==0)
          Negtive_Down_temp = 0;
          LLW_Pos_Down = -1;
          end
        state Positive_Up
          if(Positive_Up==0)
          Positive_Up_temp = 0;
          LLW_Pos_Up = 1;
          end
        state Positive_Down
          if(Positive_Down==0)
          Positive_Down_temp = 0;
          LLW_Pos_Up = -1;
          end
        (default) -> Adjust.LLW_Adjust.LLW_Pos_Adjust.LLW_Pos_Adjust
        Adjust.LLW_Adjust.LLW_Pos_Adjust.LLW_Pos_Adjust -> Adjust.LLW_Adjust.LLW_Pos_Adjust.Negtive_Up [order 4] : [(Negtive_Up_temp==0)&&(Negtive_Up>0)]{Negtive_Up_temp=1;}
        Adjust.LLW_Adjust.LLW_Pos_Adjust.LLW_Pos_Adjust -> Adjust.LLW_Adjust.LLW_Pos_Adjust.Negtive_Down [order 2] : [(Negtive_Down_temp==0)&&(Negtive_Down>0)]{Negtive_Down_temp=1;}
        Adjust.LLW_Adjust.LLW_Pos_Adjust.Negtive_Down -> Adjust.LLW_Adjust.LLW_Pos_Adjust.LLW_Pos_Adjust : [Negtive_Down_temp == 0]
        Adjust.LLW_Adjust.LLW_Pos_Adjust.Negtive_Up -> Adjust.LLW_Adjust.LLW_Pos_Adjust.LLW_Pos_Adjust : [Negtive_Up_temp == 0]
        Adjust.LLW_Adjust.LLW_Pos_Adjust.LLW_Pos_Adjust -> Adjust.LLW_Adjust.LLW_Pos_Adjust.Positive_Up [order 3] : [(Positive_Up_temp==0)&&(Positive_Up>0)]{Positive_Up_temp=1;}
        Adjust.LLW_Adjust.LLW_Pos_Adjust.LLW_Pos_Adjust -> Adjust.LLW_Adjust.LLW_Pos_Adjust.Positive_Down [order 1] : [(Positive_Down_temp==0)&&(Positive_Down>0)]{Positive_Down_temp=1;}
        Adjust.LLW_Adjust.LLW_Pos_Adjust.Positive_Up -> Adjust.LLW_Adjust.LLW_Pos_Adjust.LLW_Pos_Adjust : [Positive_Up_temp == 0]
        Adjust.LLW_Adjust.LLW_Pos_Adjust.Positive_Down -> Adjust.LLW_Adjust.LLW_Pos_Adjust.LLW_Pos_Adjust : [Positive_Down_temp == 0]
      Adjust.LLW_Adjust.LLW_Adjust -> LLW_Auto [order 4] : [ManualAuto=="LLW_Auto"]{Display_State=1;}
      LLW_Auto -> Adjust.LLW_Adjust.LLW_Adjust : [ManualAuto~="LLW_Auto"]{Display_State=4;}
      (default) -> Adjust.LLW_Adjust.LLW_Adjust
      Adjust.LLW_Adjust.LLW_Adjust -> Adjust.LLW_Adjust.LLW_Pos_Adjust [order 1] : [ManualAuto=="LLW_Manual_Pos"]
      Adjust.LLW_Adjust.LLW_Adjust -> Adjust.LLW_Adjust.LLW_Freq_Adjust [order 3] : [ManualAuto=="LLW_Manual_Freq"]
      Adjust.LLW_Adjust.LLW_Pos_Adjust -> Adjust.LLW_Adjust.LLW_Adjust : [ManualAuto~="LLW_Manual_Pos"]
      Adjust.LLW_Adjust.LLW_Freq_Adjust -> Adjust.LLW_Adjust.LLW_Adjust : [ManualAuto~="LLW_Manual_Freq"]
      Adjust.LLW_Adjust.LLW_Adjust -> Adjust.LLW_Adjust.LLW_Torque_Adjust [order 2] : [ManualAuto=="LLW_Manual_Torque"]
      Adjust.LLW_Adjust.LLW_Torque_Adjust -> Adjust.LLW_Adjust.LLW_Adjust : [ManualAuto~="LLW_Manual_Torque"]
    Adjust.Adjust -> LLF_Adjust [order 4] : [Mode=="Lower_Limb_Follow"]{Display_State=1;}
    LLF_Adjust -> Adjust.Adjust : [Mode~="Lower_Limb_Follow"]
    (default) -> Adjust.Adjust
    Adjust.Adjust -> Adjust.LLW_Adjust [order 1] : [Mode=="Lower_Limb_Walk"]{Display_State=4;}
    Adjust.Adjust -> Adjust.LLFK_Adjust [order 2] : [Mode=="Lower_Limb_FlutterKick"]{Display_State=2;}
    Adjust.LLW_Adjust -> Adjust.Adjust : [Mode~="Lower_Limb_Walk"]
    Adjust.LLFK_Adjust -> Adjust.Adjust : [Mode~="Lower_Limb_FlutterKick"]
    Adjust.LLB_Adjust -> Adjust.Adjust : [Mode~="Lower_Limb_Breaststroke"]
    Adjust.Adjust -> Adjust.LLB_Adjust [order 3] : [Mode=="Lower_Limb_Breaststroke"]{Display_State=3;}
  (default) -> Start
  Start -> Adjust : [State == "Stop"]
  Adjust -> Start : [State ~= "Stop"]
  data: kState output string; Display_State output; Freq_Up input; Freq_Down input; Positive_Up input; Positive_Down input; Negtive_Up input; Negtive_Down input; LLFK_Torque_Up output; LLFK_Torque_Down output; LLFK_Freq output; LLFK_Pos_Up output; LLFK_Pos_Down output; State input; Mode input; ManualAuto input; LLB_Freq output; LLB_Torque_Up output; LLB_Torque_Down output; LLB_Pos_Up output; LLB_Pos_Down output; LLW_Freq output; LLW_Torque_Up output; LLW_Torque_Down output; LLW_Pos_Up output; LLW_Pos_Down output; Freq_Up_temp local; Freq_Down_temp local; Positive_Up_temp local; Negtive_Up_temp local; Positive_Down_temp local; Negtive_Down_temp local

== stateflow chart TestStructure/Control/PanelController/LowerLimbTaskControlStateMachine ==
  state PauseTask
    ControlState = 9;
    ResetState = 0;
  state StopTask
    ControlState = 1;
  state StartTask
    state Start
    state LLFTask
      ControlState = 2;
    state LLFK
      state LLFK
      state LLFKManualTask
        ControlState = 3;
      state LLFKAutoTask
        ControlState = 4;
      (default) -> StartTask.LLFK.LLFK
      StartTask.LLFK.LLFK -> LLFKManualTask [order 1] : [ManualAuto~="LLFK_Auto"]
      StartTask.LLFK.LLFK -> LLFKAutoTask [order 2] : [ManualAuto=="LLFK_Auto"]
      LLFKManualTask -> StartTask.LLFK.LLFK : [ManualAuto=="LLFK_Auto"]
      LLFKAutoTask -> StartTask.LLFK.LLFK : [ManualAuto~="LLFK_Auto"]
    state LLB
      state LLB
      state LLBManualTask
        ControlState = 5;
      state LLBAutoTask
        ControlState = 6;
      (default) -> StartTask.LLB.LLB
      StartTask.LLB.LLB -> LLBAutoTask [order 2] : [ManualAuto=="LLB_Auto"]
      StartTask.LLB.LLB -> LLBManualTask [order 1] : [ManualAuto~="LLB_Auto"]
      LLBAutoTask -> StartTask.LLB.LLB : [ManualAuto~="LLB_Auto"]
      LLBManualTask -> StartTask.LLB.LLB : [ManualAuto=="LLB_Auto"]
    state LLW
      state LLW
      state LLWManualTask
        ControlState = 7;
      state LLWAutoTask
        ControlState = 8;
      (default) -> StartTask.LLW.LLW
      StartTask.LLW.LLW -> LLWManualTask [order 1] : [ManualAuto~="LLW_Auto"]
      StartTask.LLW.LLW -> LLWAutoTask [order 2] : [ManualAuto=="LLW_Auto"]
      LLWAutoTask -> StartTask.LLW.LLW : [ManualAuto~="LLW_Auto"]
      LLWManualTask -> StartTask.LLW.LLW : [ManualAuto=="LLW_Auto"]
    (default) -> Start
    Start -> LLFTask [order 1] : [Mode=="Lower_Limb_Follow"]
    Start -> StartTask.LLFK [order 2] : [Mode=="Lower_Limb_FlutterKick"]
    Start -> StartTask.LLW [order 4] : [Mode=="Lower_Limb_Walk"]
    StartTask.LLB -> Start : [Mode~="Lower_Limb_Breaststroke"]
    LLFTask -> Start : [Mode~="Lower_Limb_Follow"]
    StartTask.LLFK -> Start : [Mode~="Lower_Limb_FlutterKick"]
    StartTask.LLW -> Start : [Mode~="Lower_Limb_Walk"]
    Start -> StartTask.LLB [order 3] : [Mode=="Lower_Limb_Breaststroke"]
  (default) -> PauseTask
  PauseTask -> StartTask [order 2] : [State=="Start"]
  PauseTask -> StopTask [order 1] : [State=="Stop"]{ResetState = 1;}
  StartTask -> PauseTask : [State=="Pause"]
  StopTask -> StartTask : [State=="Start"]{ResetState = 0;}
  data: State input; Mode input; ManualAuto input; ControlState output; ResetState output

== stateflow chart TestStructure/Control/PanelController/UpperLimbTaskControlStateMachine ==
  state PauseTask
    ControlState = 1;
  state StopTask
    ControlState = 1;
  state StartTask
    state UnlockTask
      ControlState = 1;
    state LockTask
      ControlState = 2;
    (default) -> UnlockTask
    UnlockTask -> LockTask : [UnlockLock=="UpperLimb_Lock"]
    LockTask -> UnlockTask : [UnlockLock=="UpperLimb_Unlock"]
  (default) -> PauseTask
  PauseTask -> StartTask [order 2] : [State=="Start"]
  PauseTask -> StopTask [order 1] : [State=="Stop"]
  StartTask -> PauseTask : [State=="Pause"]
  StopTask -> StartTask : [State=="Start"]
  data: TaskFinished input; State input; UnlockLock input; ControlState output

== matlab function TestStructure/Control/Tasks/StopTask/MATLAB Function1 ==
  data: u input; y output; Pos input
function y = Current_P(u, Pos)
y = sign(u)*min(abs(u),abs(Pos)*0.1);

== matlab function TestStructure/Control/Tasks/StopTask/MATLAB Function2 ==
  data: u input; y output; Pos input
function y = Current_P(u, Pos)
y = sign(u)*min(abs(u),abs(Pos)*0.1);

== matlab function TestStructure/Control/Tasks/StopTask/MATLAB Function3 ==
  data: u input; y output; Pos input
function y = Current_P(u, Pos)
y = sign(u)*min(abs(u),abs(Pos)*0.1);

== matlab function TestStructure/Control/Tasks/StopTask/MATLAB Function4 ==
  data: u input; y output; Pos input
function y = Current_P(u, Pos)
y = sign(u)*min(abs(u),abs(Pos)*0.1);
